simulink model "Lock_Mode_Management"  (Simulink 7.9)
settings: Solver=FixedStepDiscrete  StartTime=0.0  StopTime=10  RelTol=1e-3  SampleTimeConstraint=STIndependent
undefined symbols (not defined in the file or in its folder): ActuatorStatus
CloseFcn:
  | rtwprivate ssgencode ModelCloseRequest ADL
settings Model: MinMaxOverflowLogging=ForceOff  Creator=fguerin  LastModifiedBy=klindqvi  CovMetricSettings=dcme  CovHtmlReporting=off  covSaveCumulativeToWorkspaceVar=off  CovSaveSingleToWorkspaceVar=off  CovModelRefEnable=off  CovExternalEMLEnable=on
settings DataIOCC: ExternalInput=[t,u]  LimitDataPoints=off  LoadExternalInput=on  SaveOutput=off  DSMLogging=off  SaveTime=off  SignalLoggingName=logsOut
settings OptimizationCC: InlineParams=on  InlineInvariantSignals=on  EnhancedBackFolding=on  ZeroExternalMemoryAtStartup=off  ZeroInternalMemoryAtStartup=off  EfficientFloat2IntCast=on  OptimizeModelRefInitCode=on  LifeSpan=1
settings DebuggingCC: ReadBeforeWriteMsg=EnableAllAsError  WriteAfterWriteMsg=EnableAllAsError  WriteAfterReadMsg=EnableAllAsError  AlgebraicLoopMsg=error  ArtificialAlgebraicLoopMsg=error  SaveWithDisabledLinksMsg=error  SaveWithParameterizedLinksMsg=error  CheckExecutionContextPreStartOutputMsg=on  CheckExecutionContextRuntimeOutputMsg=on  BlockPriorityViolationMsg=error  SolverPrmCheckMsg=error  MultiTaskCondExecSysMsg=warning  MultiTaskRateTransMsg=warning  IntegerOverflowMsg=none  ParameterUnderflowMsg=error  ParameterPrecisionLossMsg=error  ParameterTunabilityLossMsg=error  UnderSpecifiedDataTypeMsg=warning  UnnecessaryDatatypeConvMsg=warning  VectorMatrixConversionMsg=error  SignalLabelMismatchMsg=warning  SFcnCompatibilityMsg=error  BusObjectLabelMismatch=error  RootOutportRequireBusObject=error  AssertControl=DisableAll  ModelReferenceIOMsg=error  ModelReferenceIOMismatchMessage=error  ModelReferenceCSMismatchMessage=warning  UnknownTsInhSupMsg=error  ModelReferenceDataLoggingMessage=error  ModelReferenceSymbolNameMessage=none  StrictBusMsg=ErrorOnBusTreatedAsVector
settings HardwareCC: ProdLargestAtomicInteger=Long  ProdLargestAtomicFloat=Double  ProdIntDivRoundTo=Zero  ProdEndianess=BigEndian  ProdHWDeviceType=Freescale->MPC5500
settings ModelReferenceCC: ModelReferenceNumInstancesAllowed=Single
settings SFSimCC: SimParseCustomCode=off
settings RTWCC: SystemTargetFile=ert.tlc  TemplateMakefile=ert_default_tmf  Description=Embedded Coder  GenerateReport=on  RTWVerbose=off  ProcessScript=ert_make_rtw_hook  IncludeHyperlinkInReport=on  LaunchReport=on  GenerateTraceInfo=on  GenerateTraceReport=on  GenerateTraceReportSl=on  GenerateTraceReportSf=on  GenerateTraceReportEml=on  GenerateCodeMetricsReport=on
settings MATStruct: className=rtw.pil.Bullseye  argsAllComponents=[]  excludedModels=[]  includeReferencedModels=off  includeTopModel=on  enabled=on
settings CodeAppCC: ForceParamTrailComments=on  IgnoreCustomStorageClasses=off  IgnoreTestpoints=on  MangleLength=4  InlinedPrmAccess=Macros  ReqsInCode=on
settings ERTTargetCC: CodeReplacementLibrary=ANSI_C  MultiwordLength=2048  SupportAbsoluteTime=off  SupportNonFinite=off  SupportComplex=off  PortableWordSizes=on  InlinedParameterPlacement=NonHierarchical  ERTCustomFileTemplate=example_file_process.tlc  ConvertIfToSwitch=off  SuppressUnreachableDefaultCases=off
settings ConfigComp: Description=Design Verifier Custom Configuration Component  DVMaxProcessTime=600  DVDisplayUnsatisfiableObjectives=on  DVAutomaticStubbing=off  DVOutputDir=C:\Work\Data\Pilots\P_PSA_ECoder_BenchMark_LaGarenne\source9b\deliverable\trunk\demos\VnV_example\Projects\ADL_Project/Simulink_Test_Generation/ADL_Sim  DVModelCoverageObjectives=MCDC  DVTestSuiteOptimization=CombinedObjectives  DVDataFileName=./Tests/$ModelName$_sldvdata  DVSaveHarnessModel=on  DVHarnessModelFileName=./Tests/$ModelName$_testHarness  DVModelReferenceHarness=on  DVSaveReport=on  DVReportFileName=ADL_Sim_SLDV.html

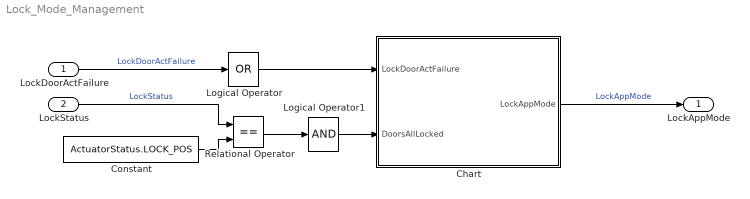
== system Lock_Mode_Management ==
  LockDoorActFailure : Inport  OutDataTypeStr=boolean  PortDimensions=2
  LockStatus : Inport  Port=2  PortDimensions=2
  Chart : Stateflow chart  TreatAsAtomicUnit=on
  Constant : Constant  Value=ActuatorStatus.LOCK_POS
  Logical Operator : Logic  Operator=OR  Inputs=1  AllPortsSameDT=off  OutDataTypeStr=boolean
  Logical Operator1 : Logic  Inputs=1  AllPortsSameDT=off  OutDataTypeStr=boolean
  Relational Operator : RelationalOperator  Operator===  OutDataTypeStr=boolean
  LockAppMode : Outport  OutDataTypeStr=Enum: LockingMode  PortDimensions=1
  wires:
  LockDoorActFailure/1 -> Logical Operator/1  "LockDoorActFailure"
  Chart/1(LockAppMode) -> LockAppMode/1  "LockAppMode"
  Logical Operator/1 -> Chart/1(LockDoorActFailure)
  LockStatus/1 -> Relational Operator/1  "LockStatus"
  Constant/1 -> Relational Operator/2
  Relational Operator/1 -> Logical Operator1/1
  Logical Operator1/1 -> Chart/2(DoorsAllLocked)

== stateflow chart Chart ==
  state Normal
    state Unlock
      entry:
      LockAppMode = ...
      LockingMode.NORMAL_UNLOCK;
    state Lock
      entry:
      LockAppMode = ...
      LockingMode.NORMAL_LOCK;
    (default) -> Unlock
    Unlock -> Lock : [DoorsAllLocked]
    Lock -> Unlock : [!DoorsAllLocked]
  state Failure
    entry:
    LockAppMode = LockingMode.FAILURE;
  (default) -> Normal
  Normal -> Failure : [LockDoorActFailure]
  data: LockDoorActFailure input double; LockAppMode output double; DoorsAllLocked input double
